simulink model "FourAGVsFullModel"  (R2019b)
settings: Solver=VariableStepAuto  StartTime=0.0  StopTime=200  RelTol=1e-3
values from neighbouring files (symbols this model uses):
  n = Datesize(1,1)    [AGVPlot.m]
undefined symbols (not defined in the file or in its folder): m, sigbuilder_block
settings Model: PacingRate=2  Creator=Khaled  LastModifiedBy=Khaled

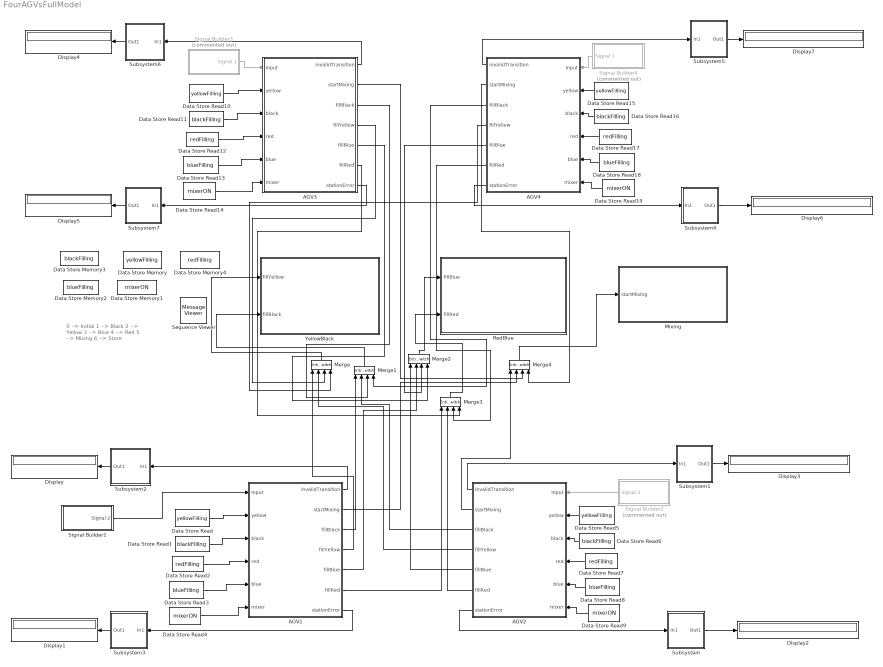
== system FourAGVsFullModel ==
  note: 0 --> Initial
      | 1 --> Black
      | 2 --> Yellow
      | 3 --> Blue
      | 4 --> Red
      | 5 --> Mixing
      | 6 --> Store
  AGV1 : Stateflow chart  BlockKeywords=__PRM__SERIALIZED__DATA__:Stateflow Chart,Stateflow Diagram  TreatAsAtomicUnit=on
  AGV2 : Stateflow chart  BlockKeywords=__PRM__SERIALIZED__DATA__:Stateflow Chart,Stateflow Diagram  TreatAsAtomicUnit=on
  AGV3 : Stateflow chart  BlockKeywords=__PRM__SERIALIZED__DATA__:Stateflow Chart,Stateflow Diagram  TreatAsAtomicUnit=on
  AGV4 : Stateflow chart  BlockKeywords=__PRM__SERIALIZED__DATA__:Stateflow Chart,Stateflow Diagram  TreatAsAtomicUnit=on
  Data Store Read{,5,10,15} (4 alike) : DataStoreRead  DataStoreName=yellowFilling
  Data Store Read{1,6,11,16} (4 alike) : DataStoreRead  DataStoreName=blackFilling
  Data Store Read{2,7,12,17} (4 alike) : DataStoreRead  DataStoreName=redFilling
  Data Store Read{3,8,13,18} (4 alike) : DataStoreRead  DataStoreName=blueFilling
  Data Store Read{4,9,14,19} (4 alike) : DataStoreRead  DataStoreName=mixerON
  Data Store Memory : DataStoreMemory  DataStoreName=yellowFilling  ReadBeforeWriteMsg=warning  WriteAfterWriteMsg=warning  WriteAfterReadMsg=warning  ShowAdditionalParam=off  OutDataTypeStr=double
  Data Store Memory1 : DataStoreMemory  DataStoreName=mixerON  ReadBeforeWriteMsg=warning  WriteAfterWriteMsg=warning  WriteAfterReadMsg=warning  ShowAdditionalParam=off  OutDataTypeStr=double
  Data Store Memory2 : DataStoreMemory  DataStoreName=blueFilling  ReadBeforeWriteMsg=warning  WriteAfterWriteMsg=warning  WriteAfterReadMsg=warning  ShowAdditionalParam=off  OutDataTypeStr=double
  Data Store Memory3 : DataStoreMemory  DataStoreName=blackFilling  ReadBeforeWriteMsg=warning  WriteAfterWriteMsg=warning  WriteAfterReadMsg=warning  ShowAdditionalParam=off  OutDataTypeStr=double
  Data Store Memory4 : DataStoreMemory  DataStoreName=redFilling  ReadBeforeWriteMsg=warning  WriteAfterWriteMsg=warning  WriteAfterReadMsg=warning  ShowAdditionalParam=off  OutDataTypeStr=double
  Display{,1..7} (8 alike) : Display
  Merge{,1..4} (5 alike) : EntityInputSwitch  InputPortMessageModes=m,m,m,m  OutputPortMessageModes=m  NumberInputPorts=4  SwitchingCriterion=From control port  InitialPortSelection=x
      settings: InputPortMap=u1,u2,u3,u4
  Mixing : Stateflow chart  BlockKeywords=__PRM__SERIALIZED__DATA__:Stateflow Chart,Stateflow Diagram  TreatAsAtomicUnit=on
  RedBlue : Stateflow chart  BlockKeywords=__PRM__SERIALIZED__DATA__:Stateflow Chart,Stateflow Diagram  TreatAsAtomicUnit=on
  Sequence Viewer : MessageViewer  VariableStepTimePrecision=16  ShowAllLifelines=off  AutoLayout=off  History=100  ShowMessages=off
  Signal Builder1 : Subsystem  Tag=STV Subsys  LoadFcn=sigbuilder_block('load');  StartFcn=sigbuilder_block('start');  StopFcn=sigbuilder_block('stop');  ClipboardFcn=sigbuilder_block('clipboard');  mask(Sigbuilder block){tuvar=[0:10]}
      mask help: Simulink:masks:SigbuilderBlock_MD
      mask init:
      | if ~strcmp(get_param(bdroot(gcbh),'SimulationStatus'),'stopped') tuvar = sigbuilder_block('maskInit'); end
      settings: CopyFcn=sigbuilder_block('copy');  DeleteFcn=sigbuilder_block('delete');  ModelCloseFcn=sigbuilder_block('modelClose');  PreSaveFcn=sigbuilder_block('preSave');  PauseFcn=sigbuilder_block('pause');  ContinueFcn=sigbuilder_block('continue');  NameChangeFcn=sigbuilder_block('namechange');  OpenFcn=sigbuilder_block('open',[5.4 30 1141.2 522.6 ]);  CloseFcn=sigbuilder_block('close');
      mask Display: plot(0, 0, 100, 100,[2, 2, 32, 32, 2], [68, 8, 8, 68, 68],[32, 2], [38, 38], [32, 19, 2],[53, 60, 44], [32, 17, 17, 2],[16, 16, 31, 31]);txt = getActiveGroup(gcbh);text(2, 100, txt,'verticalAlignment', 'top');
  Signal Builder2 : Subsystem  Tag=STV Subsys  Commented=on  LoadFcn=sigbuilder_block('load');  StartFcn=sigbuilder_block('start');  StopFcn=sigbuilder_block('stop');  ClipboardFcn=sigbuilder_block('clipboard');  mask(Sigbuilder block){tuvar=[0:10]}
      mask help: Simulink:masks:SigbuilderBlock_MD
      mask init:
      | if ~strcmp(get_param(bdroot(gcbh),'SimulationStatus'),'stopped') tuvar = sigbuilder_block('maskInit'); end
      settings: CopyFcn=sigbuilder_block('copy');  DeleteFcn=sigbuilder_block('delete');  ModelCloseFcn=sigbuilder_block('modelClose');  PreSaveFcn=sigbuilder_block('preSave');  PauseFcn=sigbuilder_block('pause');  ContinueFcn=sigbuilder_block('continue');  NameChangeFcn=sigbuilder_block('namechange');  OpenFcn=sigbuilder_block('open',[-61.2 14.4 1141.2 522.6 ]);  CloseFcn=sigbuilder_block('close');
      mask Display: plot(0, 0, 100, 100,[2, 2, 32, 32, 2], [68, 8, 8, 68, 68],[32, 2], [38, 38], [32, 19, 2],[53, 60, 44], [32, 17, 17, 2],[16, 16, 31, 31]);txt = getActiveGroup(gcbh);text(2, 100, txt,'verticalAlignment', 'top');
  Signal Builder3 : Subsystem  Tag=STV Subsys  Commented=on  LoadFcn=sigbuilder_block('load');  StartFcn=sigbuilder_block('start');  StopFcn=sigbuilder_block('stop');  ClipboardFcn=sigbuilder_block('clipboard');  mask(Sigbuilder block){tuvar=[0:10]}
      mask help: Simulink:masks:SigbuilderBlock_MD
      mask init:
      | if ~strcmp(get_param(bdroot(gcbh),'SimulationStatus'),'stopped') tuvar = sigbuilder_block('maskInit'); end
      settings: CopyFcn=sigbuilder_block('copy');  DeleteFcn=sigbuilder_block('delete');  ModelCloseFcn=sigbuilder_block('modelClose');  PreSaveFcn=sigbuilder_block('preSave');  PauseFcn=sigbuilder_block('pause');  ContinueFcn=sigbuilder_block('continue');  NameChangeFcn=sigbuilder_block('namechange');  OpenFcn=sigbuilder_block('open',[303.6 76.2 579.6 400.2 ]);  CloseFcn=sigbuilder_block('close');
      mask Display: plot(0, 0, 100, 100,[2, 2, 32, 32, 2], [68, 8, 8, 68, 68],[32, 2], [38, 38], [32, 19, 2],[53, 60, 44], [32, 17, 17, 2],[16, 16, 31, 31]);txt = getActiveGroup(gcbh);text(2, 100, txt,'verticalAlignment', 'top');
  Signal Builder4 : Subsystem  Tag=STV Subsys  Commented=on  LoadFcn=sigbuilder_block('load');  StartFcn=sigbuilder_block('start');  StopFcn=sigbuilder_block('stop');  ClipboardFcn=sigbuilder_block('clipboard');  mask(Sigbuilder block){tuvar=[0:10]}
      mask help: Simulink:masks:SigbuilderBlock_MD
      mask init:
      | if ~strcmp(get_param(bdroot(gcbh),'SimulationStatus'),'stopped') tuvar = sigbuilder_block('maskInit'); end
      settings: CopyFcn=sigbuilder_block('copy');  DeleteFcn=sigbuilder_block('delete');  ModelCloseFcn=sigbuilder_block('modelClose');  PreSaveFcn=sigbuilder_block('preSave');  PauseFcn=sigbuilder_block('pause');  ContinueFcn=sigbuilder_block('continue');  NameChangeFcn=sigbuilder_block('namechange');  OpenFcn=sigbuilder_block('open',[440.4 98.4 579.6 400.2 ]);  CloseFcn=sigbuilder_block('close');
      mask Display: plot(0, 0, 100, 100,[2, 2, 32, 32, 2], [68, 8, 8, 68, 68],[32, 2], [38, 38], [32, 19, 2],[53, 60, 44], [32, 17, 17, 2],[16, 16, 31, 31]);txt = getActiveGroup(gcbh);text(2, 100, txt,'verticalAlignment', 'top');
  Subsystem : Subsystem
  Subsystem1 : Subsystem
  Subsystem2 : Subsystem
  Subsystem3 : Subsystem
  Subsystem4 : Subsystem
  Subsystem5 : Subsystem
  Subsystem6 : Subsystem
  Subsystem7 : Subsystem
  YellowBlack : Stateflow chart  BlockKeywords=__PRM__SERIALIZED__DATA__:Stateflow Chart,Stateflow Diagram  TreatAsAtomicUnit=on
  wires:
  AGV3/6(fillRed) -> Merge3/4
  Data Store Read5/1 -> AGV2/2(yellow)
  Data Store Read18/1 -> AGV4/5(blue)
  AGV3/2(startMixing) -> Merge4/3
  AGV3/1(invalidTransition) -> Subsystem6/1(In1)
  Data Store Read6/1 -> AGV2/3(black)
  AGV3/3(fillBlack) -> Merge1/3
  Data Store Read19/1 -> AGV4/6(mixer)
  Data Store Read14/1 -> AGV3/6(mixer)
  Data Store Read12/1 -> AGV3/4(red)
  AGV4/2(startMixing) -> Merge4/4
  Subsystem5/1(Out1) -> Display7/1
  AGV3/4(fillYellow) -> Merge/3
  Merge4/1 -> Mixing/1(startMixing)
  AGV3/7(stationError) -> Subsystem7/1(In1)
  Data Store Read8/1 -> AGV2/5(blue)
  Data Store Read13/1 -> AGV3/5(blue)
  Signal Builder3/1(Signal 1) -> AGV3/1(Input)
  AGV1/6(fillRed) -> Merge3/1
  AGV4/7(stationError) -> Subsystem4/1(In1)
  Data Store Read11/1 -> AGV3/3(black)
  Subsystem7/1(Out1) -> Display5/1
  Signal Builder4/1(Signal 1) -> AGV4/1(Input)
  Subsystem4/1(Out1) -> Display6/1
  AGV3/5(fillBlue) -> Merge2/4
  Data Store Read4/1 -> AGV1/6(mixer)
  Data Store Read17/1 -> AGV4/4(red)
  Data Store Read16/1 -> AGV4/3(black)
  AGV2/2(startMixing) -> Merge4/1
  AGV4/6(fillRed) -> Merge3/3
  Data Store Read15/1 -> AGV4/2(yellow)
  AGV1/1(invalidTransition) -> Subsystem2/1(In1)
  Data Store Read7/1 -> AGV2/4(red)
  Signal Builder2/1(Signal 2) -> AGV2/1(Input)
  AGV2/1(invalidTransition) -> Subsystem1/1(In1)
  Subsystem1/1(Out1) -> Display3/1
  AGV2/7(stationError) -> Subsystem/1(In1)
  Subsystem6/1(Out1) -> Display4/1
  Subsystem3/1(Out1) -> Display1/1
  AGV4/5(fillBlue) -> Merge2/3
  AGV2/5(fillBlue) -> Merge2/1
  AGV1/7(stationError) -> Subsystem3/1(In1)
  AGV1/5(fillBlue) -> Merge2/2
  Subsystem2/1(Out1) -> Display/1
  Data Store Read10/1 -> AGV3/2(yellow)
  Data Store Read1/1 -> AGV1/3(black)
  AGV1/3(fillBlack) -> Merge1/1
  Data Store Read9/1 -> AGV2/6(mixer)
  Merge3/1 -> RedBlue/2(fillRed)
  Merge/1 -> YellowBlack/1(fillYellow)
  AGV1/2(startMixing) -> Merge4/2
  AGV4/3(fillBlack) -> Merge1/4
  AGV2/3(fillBlack) -> Merge1/2
  AGV4/1(invalidTransition) -> Subsystem5/1(In1)
  Merge1/1 -> YellowBlack/2(fillBlack)
  Merge2/1 -> RedBlue/1(fillBlue)
  AGV2/6(fillRed) -> Merge3/2
  AGV4/4(fillYellow) -> Merge/4
  Data Store Read/1 -> AGV1/2(yellow)
  Data Store Read3/1 -> AGV1/5(blue)
  AGV2/4(fillYellow) -> Merge/2
  Subsystem/1(Out1) -> Display2/1
  AGV1/4(fillYellow) -> Merge/1
  Data Store Read2/1 -> AGV1/4(red)
  Signal Builder1/1(Signal 2) -> AGV1/1(Input)

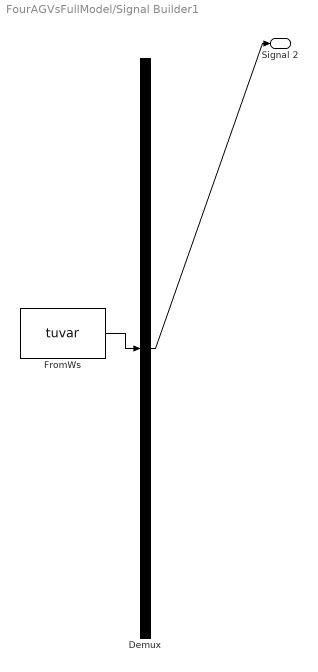
== system FourAGVsFullModel/Signal Builder1 ==
  Demux : Demux  Tag=STV Demux  Outputs=1
  FromWs : FromWorkspace  Tag=STV FromWs  VariableName=tuvar  SampleTime=0
      SigBuilderData=|
      | common.afterFinalStr = 'Extrapolate'
      | common.sampleTime = 0
      | dataSet.timeRange = [0 345]
      | dataSet.name = 'Group 1'
      | sbobj.Groups.Name = 'Group 1'
      | sbobj.Groups.Signals.Name = 'Signal 2'
      | sbobj.Groups.Signals.XData = [0 30 30 60 60 80 80 105 105 150 150 185 185 195 195 225 225 245 245 300 300 309.5 314.5 317 320.5 325 329 333 335 335 338.5 341.5 345]
      | sbobj.Groups.Signals.YData = [0 0 6 6 1 1 3 3 5 5 6 6 0 0 6 6 2 2 5 5 6 6 6 6 6 6 6 6 6 0 0 0 0]
      | sbobj.Groups.TimeRange = [0 345]
  Signal 2 : Outport  Tag=STV Outport
  wires:
  FromWs/1 -> Demux/1
  Demux/1 -> Signal 2/1

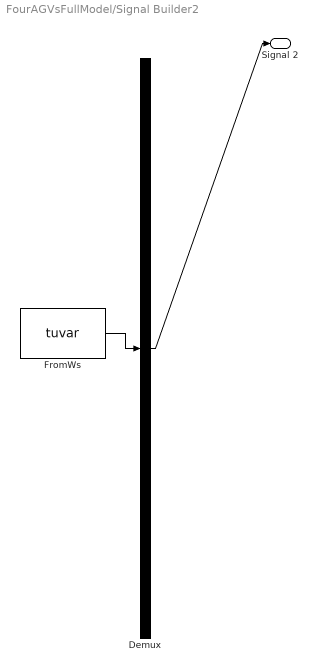
== system FourAGVsFullModel/Signal Builder2 ==
  Demux : Demux  Tag=STV Demux  Outputs=1
  FromWs : FromWorkspace  Tag=STV FromWs  VariableName=tuvar  SampleTime=0
      SigBuilderData=|
      | common.afterFinalStr = 'Extrapolate'
      | common.sampleTime = 0
      | dataSet.timeRange = [0 400]
      | dataSet.name = 'Group 1'
      | sbobj.Groups.Name = 'Group 1'
      | sbobj.Groups.Signals.Name = 'Signal 2'
      | sbobj.Groups.Signals.XData = [0 30 30 50 50 75 75 110 110 120 120 150 150 180 180 225 225 260 260 270 270 300 300 320 320 332 340 345 345 358 366 371.5 380 380 400]
      | sbobj.Groups.Signals.YData = [6 6 3 3 5 5 6 6 0 0 6 6 2 2 5 5 6 6 0 0 6 6 4 4 5 5 5 5 6 6 6 6 6 0 0]
      | sbobj.Groups.TimeRange = [0 400]
  Signal 2 : Outport  Tag=STV Outport
  wires:
  FromWs/1 -> Demux/1
  Demux/1 -> Signal 2/1

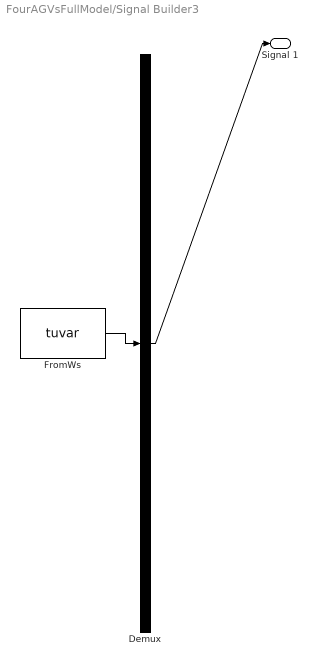
== system FourAGVsFullModel/Signal Builder3 ==
  Demux : Demux  Tag=STV Demux  Outputs=1
  FromWs : FromWorkspace  Tag=STV FromWs  VariableName=tuvar  SampleTime=0
      SigBuilderData=|
      | common.afterFinalStr = 'Extrapolate'
      | common.sampleTime = 0
      | dataSet.timeRange = [0 100]
      | dataSet.name = 'Group 1'
      | sbobj.Groups.Name = 'Group 1'
      | sbobj.Groups.Signals.Name = 'Signal 1'
      | sbobj.Groups.Signals.XData = [0 23 23 46 46 66 66 87.5 87.5 93.75 100]
      | sbobj.Groups.Signals.YData = [2 2 4 4 5 5 6 6 0 0 0]
      | sbobj.Groups.TimeRange = [0 100]
  Signal 1 : Outport  Tag=STV Outport
  wires:
  FromWs/1 -> Demux/1
  Demux/1 -> Signal 1/1

== system FourAGVsFullModel/Signal Builder4 ==
  Demux : Demux  Tag=STV Demux  Outputs=1
  FromWs : FromWorkspace  Tag=STV FromWs  VariableName=tuvar  SampleTime=0
      SigBuilderData=|
      | common.afterFinalStr = 'Extrapolate'
      | common.sampleTime = 0
      | dataSet.timeRange = [0 100]
      | dataSet.name = 'Group 1'
      | sbobj.Groups.Name = 'Group 1'
      | sbobj.Groups.Signals.Name = 'Signal 1'
      | sbobj.Groups.Signals.XData = [0 23 23 46 66 66 87.5 87.5 93.75 100]
      | sbobj.Groups.Signals.YData = [0 0 4 4 4 5 5 0 0 0]
      | sbobj.Groups.TimeRange = [0 100]
  Signal 1 : Outport  Tag=STV Outport
  wires:
  FromWs/1 -> Demux/1
  Demux/1 -> Signal 1/1

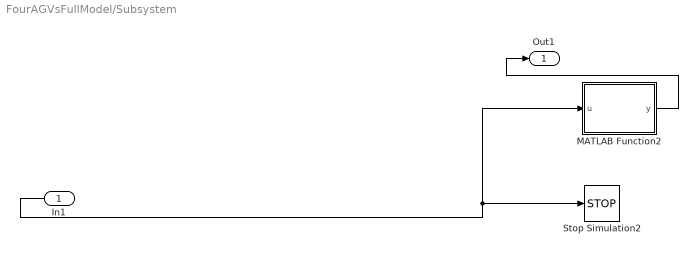
== system FourAGVsFullModel/Subsystem ==
  In1 : Inport
  MATLAB Function2 : MATLAB Function  TreatAsAtomicUnit=on
  Stop Simulation2 : Stop
  Out1 : Outport
  wires:
  In1/1 -> MATLAB Function2/1(u), Stop Simulation2/1
  MATLAB Function2/1(y) -> Out1/1

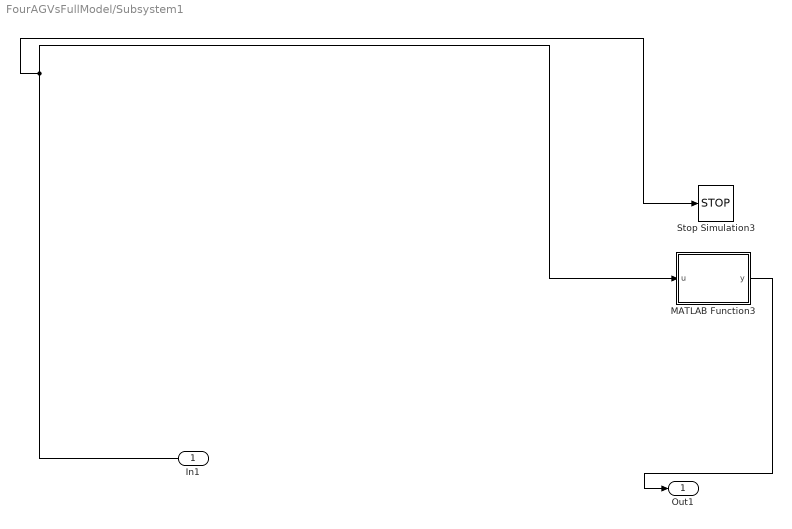
== system FourAGVsFullModel/Subsystem1 ==
  In1 : Inport
  MATLAB Function3 : MATLAB Function  TreatAsAtomicUnit=on
  Stop Simulation3 : Stop
  Out1 : Outport
  wires:
  In1/1 -> Stop Simulation3/1, MATLAB Function3/1(u)
  MATLAB Function3/1(y) -> Out1/1

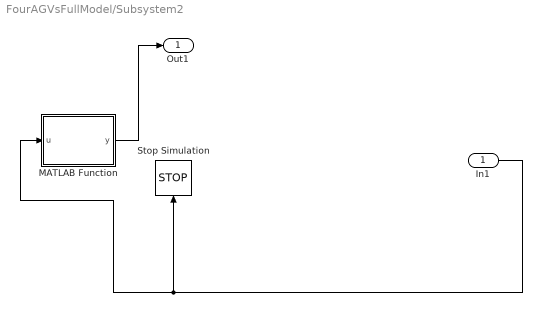
== system FourAGVsFullModel/Subsystem2 ==
  In1 : Inport
  MATLAB Function : MATLAB Function  TreatAsAtomicUnit=on
  Stop Simulation : Stop
  Out1 : Outport
  wires:
  MATLAB Function/1(y) -> Out1/1
  In1/1 -> MATLAB Function/1(u), Stop Simulation/1

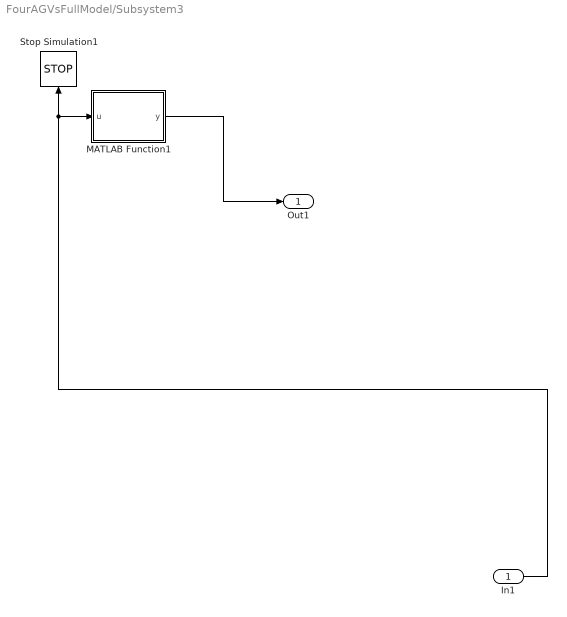
== system FourAGVsFullModel/Subsystem3 ==
  In1 : Inport
  MATLAB Function1 : MATLAB Function  TreatAsAtomicUnit=on
  Stop Simulation1 : Stop
  Out1 : Outport
  wires:
  In1/1 -> Stop Simulation1/1, MATLAB Function1/1(u)
  MATLAB Function1/1(y) -> Out1/1

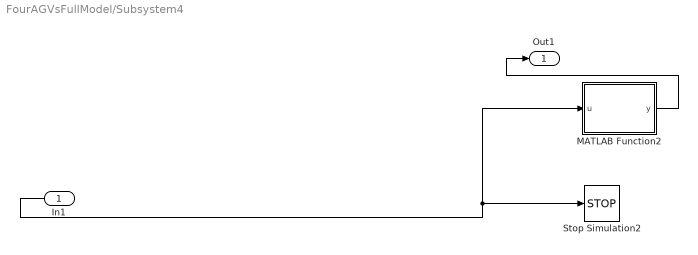
== system FourAGVsFullModel/Subsystem4 ==
  In1 : Inport
  MATLAB Function2 : MATLAB Function  TreatAsAtomicUnit=on
  Stop Simulation2 : Stop
  Out1 : Outport
  wires:
  In1/1 -> MATLAB Function2/1(u), Stop Simulation2/1
  MATLAB Function2/1(y) -> Out1/1

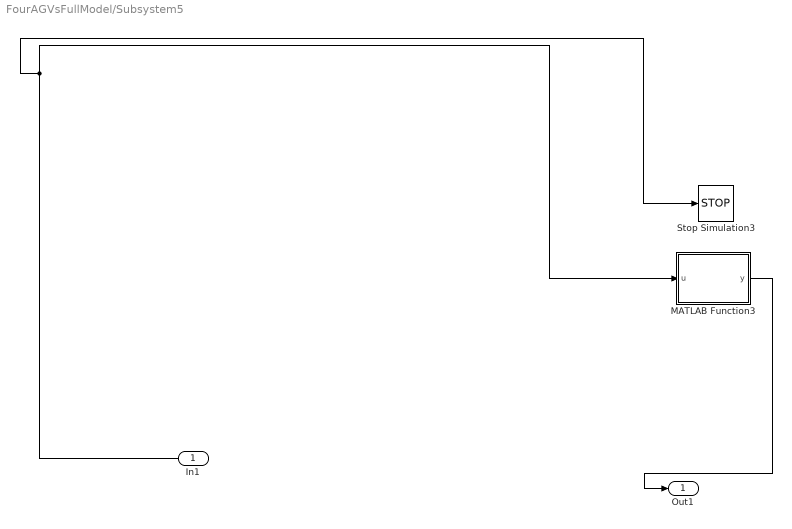
== system FourAGVsFullModel/Subsystem5 ==
  In1 : Inport
  MATLAB Function3 : MATLAB Function  TreatAsAtomicUnit=on
  Stop Simulation3 : Stop
  Out1 : Outport
  wires:
  In1/1 -> Stop Simulation3/1, MATLAB Function3/1(u)
  MATLAB Function3/1(y) -> Out1/1

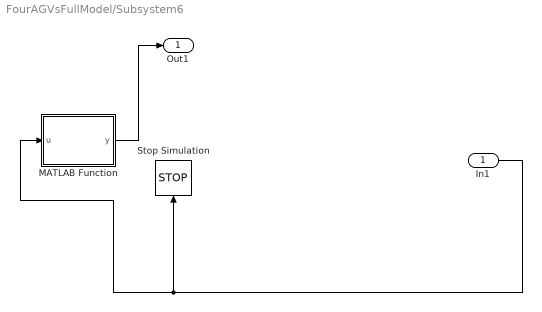
== system FourAGVsFullModel/Subsystem6 ==
  In1 : Inport
  MATLAB Function : MATLAB Function  TreatAsAtomicUnit=on
  Stop Simulation : Stop
  Out1 : Outport
  wires:
  MATLAB Function/1(y) -> Out1/1
  In1/1 -> MATLAB Function/1(u), Stop Simulation/1

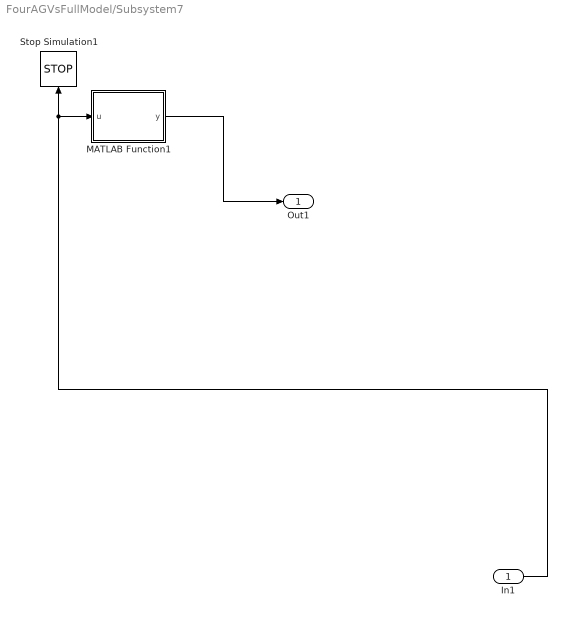
== system FourAGVsFullModel/Subsystem7 ==
  In1 : Inport
  MATLAB Function1 : MATLAB Function  TreatAsAtomicUnit=on
  Stop Simulation1 : Stop
  Out1 : Outport
  wires:
  In1/1 -> Stop Simulation1/1, MATLAB Function1/1(u)
  MATLAB Function1/1(y) -> Out1/1

== stateflow chart FourAGVsFullModel/AGV1 ==
  state Black
    en:
    send(fillBlack);
  state Yellow
    en:
    send(fillYellow);
  state YBToMixing
  state YBToRB
  state StorageToYB
  state StationErrorState
    stationError=1;
  state MixingStation
    en:
    send(startMixing);
  state Storage
  state InvalidTransitionState
    invalidTransition=1;
  state StorageToInit
  state InitToStorage
  state MixingToStorage
  state InitPosition
  state RBToYB
  state RBToMixing
  state StorageToRB
  state Red
    en:
    send(fillRed);
  state Blue
    en:
    send(fillBlue);
  Yellow -> YBToMixing [order 4] : [Input==5]
  Yellow -> YBToRB [order 3] : [Input==3 || Input==4]
  Yellow -> Black [order 1] : [Input==1]
  (junction 173) -> Yellow [order 1] : [black==0 && yellow==0]
  StorageToYB -> (junction 173) [order 2] : [Input==2 && after(T_S_YB,sec)]
  Black -> Yellow [order 1] : [Input==2]
  RBToYB -> (junction 173) [order 1] : [Input==2 && ...
      | after(T_RB_YB,sec)]
  (junction 173) -> StationErrorState [order 2] : [black==1 || yellow==1]
  StorageToYB -> (junction 176) [order 1] : [Input==1 && ...
      | after(T_S_YB,sec)]
  (junction 176) -> Black [order 1] : [black==0 && yellow==0]
  Black -> YBToMixing [order 4] : [Input==5]
  RBToYB -> (junction 176) [order 2] : [Input==1 && ...
      | after(T_RB_YB,sec)]
  Black -> InvalidTransitionState [order 3] : [Input==6 || Input==0]
  Black -> YBToRB [order 2] : [Input==3 || Input==4]
  Yellow -> InvalidTransitionState [order 2] : [Input==6 || Input==0]
  (junction 176) -> StationErrorState [order 2] : [black==1 || yellow==1]
  YBToMixing -> (junction 185) : [Input==5 && after(T_YB_M,sec)]
  YBToRB -> (junction 182) [order 2] : [Input==4 && ...
      | after(T_YB_RB,sec)]
  YBToRB -> (junction 179) [order 1] : [Input==3 && ...
      | after(T_YB_RB,sec)]
  Storage -> Storage [order 5] : [Input==6]
  Storage -> StorageToYB [order 1] : [Input==1 || Input==2]
  (junction 185) -> MixingStation [order 1] : [mixer==0]
  (junction 185) -> StationErrorState [order 2] : [mixer==1]
  Storage -> StorageToRB [order 3] : [Input==3 || Input==4]
  (junction 182) -> StationErrorState [order 2] : [blue==1 || red==1]
  RBToMixing -> (junction 185) : [Input==5 && ...
      |  after(T_RB_M,sec)]
  Storage -> InvalidTransitionState [order 4] : [Input==5]
  (junction 179) -> StationErrorState [order 2] : [blue==1 || red==1]
  MixingStation -> InvalidTransitionState [order 1] : [Input==0 ||Input==1 ||Input==2 ...
      | || Input==3 ||Input==4 ]
  InitToStorage -> Storage : after(T_Init_S,sec)
  MixingStation -> MixingToStorage [order 2] : [Input==6]
  MixingToStorage -> Storage : [Input==6 && after(T_M_S,sec)]
  Storage -> StorageToInit [order 2] : [Input==0]
  InitPosition -> InvalidTransitionState [order 3] : [Input==5 ]
  Red -> InvalidTransitionState [order 2] : [Input==6 || Input==0]
  Blue -> InvalidTransitionState [order 3] : [Input==6 || Input==0]
  StorageToInit -> InitPosition : after(T_Init_S,sec)
  InitPosition -> InitToStorage [order 1] : [Input==1 || Input==2 || Input==3 || Input==4|| Input==6]
  (default) -> InitPosition
  Red -> RBToYB [order 4] : [Input==2 || Input==1]
  Blue -> RBToYB [order 2] : [Input==1 || Input==2]
  InitPosition -> InitPosition [order 2] : [Input==0]
  StorageToRB -> StorageToRB [order 3] : [Input==3 || Input==4]
  Blue -> RBToMixing [order 4] : [Input==5]
  Red -> RBToMixing [order 3] : [Input==5]
  StorageToRB -> (junction 182) [order 2] : [Input==4 &&...
      |  after(T_S_RB,sec)]
  (junction 182) -> Red [order 1] : [blue==0&&red==0]
  StorageToRB -> (junction 179) [order 1] : [Input==3 && after(T_S_RB,sec)]
  (junction 179) -> Blue [order 1] : [blue==0&&red==0]
  Blue -> Red [order 1] : [Input==4]
  Red -> Blue [order 1] : [Input==3]
  data: Input input; invalidTransition output; startMixing output boolean size=1; fillBlack output boolean size=1; fillYellow output boolean size=1; fillBlue output boolean size=1; fillRed output boolean size=1; yellow input; black input; red input; blue input; mixer input; stationError output; T_YB_M constant double =10; T_RB_YB constant double =15; T_RB_M constant double =10; T_S_YB constant double =10; T_S_RB constant double =10; T_YB_RB constant double =15; T_M_S constant double =15; T_Init_S constant double =10

== matlab function FourAGVsFullModel/Subsystem2/MATLAB Function ==
  data: u input; y output string
function y= fcn(u)
if(u==1)
    y="Invalid Transition";
else
    y="No Error";
end

== stateflow chart FourAGVsFullModel/Mixing ==
  state MixerOFF
    mixerON=0;
  state MixerON
    mixerON=1;
  MixerOFF -> MixerON : startMixing
  (default) -> MixerOFF
  MixerON -> MixerOFF : after(15,sec)
  data: startMixing input; mixerON data_store_memory

== matlab function FourAGVsFullModel/Subsystem3/MATLAB Function1 ==
  data: u input; y output string
function y= fcn(u)
if(u==1)
    y="station is busy";
else
    y="No Error";
end

== stateflow chart FourAGVsFullModel/YellowBlack ==
  state Nofilling
    yellowFilling=0;
    blackFilling=0;
  state fillingBlack
    blackFilling=1;
  state FillingYellow
    yellowFilling=1;
  (default) -> Nofilling
  Nofilling -> fillingBlack [order 1] : fillBlack
  Nofilling -> FillingYellow [order 2] : fillYellow
  fillingBlack -> Nofilling : after(10,sec)
  FillingYellow -> Nofilling : after(10,sec)
  data: fillYellow input; fillBlack input; yellowFilling data_store_memory; blackFilling data_store_memory

== stateflow chart FourAGVsFullModel/RedBlue ==
  state Nofilling
    blueFilling=0;
    redFilling=0;
  state FillingRed
    redFilling=1;
  state FillingBlue
    blueFilling=1;
  (default) -> Nofilling
  Nofilling -> FillingRed [order 1] : fillRed
  Nofilling -> FillingBlue [order 2] : fillBlue
  FillingRed -> Nofilling : after(10,sec)
  FillingBlue -> Nofilling : after(10,sec)
  data: fillBlue input; fillRed input; blueFilling data_store_memory; redFilling data_store_memory

== stateflow chart FourAGVsFullModel/AGV2 ==
  state Black
    en:
    send(fillBlack);
  state Yellow
    en:
    send(fillYellow);
  state YBToMixing
  state YBToRB
  state StorageToYB
  state StationErrorState
    stationError=1;
  state MixingStation
    en:
    send(startMixing);
  state Storage
  state InvalidTransitionState
    invalidTransition=1;
  state StorageToInit
  state InitToStorage
  state MixingToStorage
  state InitPosition
  state RBToYB
  state RBToMixing
  state StorageToRB
  state Red
    en:
    send(fillRed);
  state Blue
    en:
    send(fillBlue);
  Yellow -> YBToMixing [order 4] : [Input==5]
  Yellow -> YBToRB [order 3] : [Input==3 || Input==4]
  Yellow -> Black [order 1] : [Input==1]
  (junction 173) -> Yellow [order 1] : [black==0 && yellow==0]
  StorageToYB -> (junction 173) [order 2] : [Input==2 && after(T_S_YB,sec)]
  Black -> Yellow [order 1] : [Input==2]
  RBToYB -> (junction 173) [order 1] : [Input==2 && ...
      | after(T_RB_YB,sec)]
  (junction 173) -> StationErrorState [order 2] : [black==1 || yellow==1]
  StorageToYB -> (junction 176) [order 1] : [Input==1 && ...
      | after(T_S_YB,sec)]
  (junction 176) -> Black [order 1] : [black==0 && yellow==0]
  Black -> YBToMixing [order 4] : [Input==5]
  RBToYB -> (junction 176) [order 2] : [Input==1 && ...
      | after(T_RB_YB,sec)]
  Black -> InvalidTransitionState [order 3] : [Input==6 || Input==0]
  Black -> YBToRB [order 2] : [Input==3 || Input==4]
  Yellow -> InvalidTransitionState [order 2] : [Input==6 || Input==0]
  (junction 176) -> StationErrorState [order 2] : [black==1 || yellow==1]
  YBToMixing -> (junction 185) : [Input==5 && after(T_YB_M,sec)]
  YBToRB -> (junction 182) [order 2] : [Input==4 && ...
      | after(T_YB_RB,sec)]
  YBToRB -> (junction 179) [order 1] : [Input==3 && ...
      | after(T_YB_RB,sec)]
  Storage -> Storage [order 5] : [Input==6]
  Storage -> StorageToYB [order 1] : [Input==1 || Input==2]
  (junction 185) -> MixingStation [order 1] : [mixer==0]
  (junction 185) -> StationErrorState [order 2] : [mixer==1]
  Storage -> StorageToRB [order 3] : [Input==3 || Input==4]
  (junction 182) -> StationErrorState [order 2] : [blue==1 || red==1]
  RBToMixing -> (junction 185) : [Input==5 && ...
      |  after(T_RB_M,sec)]
  Storage -> InvalidTransitionState [order 4] : [Input==5]
  (junction 179) -> StationErrorState [order 2] : [blue==1 || red==1]
  MixingStation -> InvalidTransitionState [order 1] : [Input==0 ||Input==1 ||Input==2 ...
      | || Input==3 ||Input==4 ]
  InitToStorage -> Storage : after(T_Init_S,sec)
  MixingStation -> MixingToStorage [order 2] : [Input==6]
  MixingToStorage -> Storage : [Input==6 && after(T_M_S,sec)]
  Storage -> StorageToInit [order 2] : [Input==0]
  InitPosition -> InvalidTransitionState [order 3] : [Input==5 ]
  Red -> InvalidTransitionState [order 2] : [Input==6 || Input==0]
  Blue -> InvalidTransitionState [order 3] : [Input==6 || Input==0]
  StorageToInit -> InitPosition : after(T_Init_S,sec)
  InitPosition -> InitToStorage [order 1] : [Input==1 || Input==2 || Input==3 || Input==4|| Input==6]
  (default) -> InitPosition
  Red -> RBToYB [order 4] : [Input==2 || Input==1]
  Blue -> RBToYB [order 2] : [Input==1 || Input==2]
  InitPosition -> InitPosition [order 2] : [Input==0]
  Blue -> RBToMixing [order 4] : [Input==5]
  Red -> RBToMixing [order 3] : [Input==5]
  StorageToRB -> (junction 182) [order 2] : [Input==4 &&...
      |  after(T_S_RB,sec)]
  (junction 182) -> Red [order 1] : [blue==0&&red==0]
  StorageToRB -> (junction 179) [order 1] : [Input==3 && after(T_S_RB,sec)]
  (junction 179) -> Blue [order 1] : [blue==0&&red==0]
  Blue -> Red [order 1] : [Input==4]
  Red -> Blue [order 1] : [Input==3]
  data: Input input; invalidTransition output; startMixing output boolean size=1; fillBlack output boolean size=1; fillYellow output boolean size=1; fillBlue output boolean size=1; fillRed output boolean size=1; yellow input; black input; red input; blue input; mixer input; stationError output; T_YB_M constant double =10; T_RB_YB constant double =15; T_RB_M constant double =10; T_S_YB constant double =10; T_S_RB constant double =10; T_YB_RB constant double =15; T_M_S constant double =15; T_Init_S constant double =10

== matlab function FourAGVsFullModel/Subsystem/MATLAB Function2 ==
  data: u input; y output string
function y= fcn(u)
if(u==1)
    y="station is busy";
else
    y="No Error";
end

== matlab function FourAGVsFullModel/Subsystem1/MATLAB Function3 ==
  data: u input; y output string
function y= fcn(u)
if(u==1)
    y="station is busy";
else
    y="No Error";
end

== stateflow chart FourAGVsFullModel/AGV3 ==
  state Black
    en:
    send(fillBlack);
  state Yellow
    en:
    send(fillYellow);
  state YBToMixing
  state YBToRB
  state StorageToYB
  state StationErrorState
    stationError=1;
  state MixingStation
    en:
    send(startMixing);
  state Storage
  state Transition
  state InvalidTransitionState
    invalidTransition=1;
  state StorageToInit
  state MixingToStorage
  state InitPosition
  state RBToYB
  state RBToMixing
  state StorageToRB
  state Red
    en:
    send(fillRed);
  state Blue
    en:
    send(fillBlue);
  Yellow -> YBToMixing [order 4] : [Input==5]
  Yellow -> YBToRB [order 3] : [Input==3 || Input==4]
  Yellow -> Black [order 1] : [Input==1]
  (junction 173) -> Yellow [order 1] : [black==0 && yellow==0]
  StorageToYB -> (junction 173) [order 2] : [Input==2 && after(T_S_YB,sec)]
  Black -> Yellow [order 1] : [Input==2]
  RBToYB -> (junction 173) [order 1] : [Input==2 && ...
      | after(T_RB_YB,sec)]
  (junction 173) -> StationErrorState [order 2] : [black==1 || yellow==1]
  StorageToYB -> (junction 176) [order 1] : [Input==1 && ...
      | after(T_S_YB,sec)]
  (junction 176) -> Black [order 1] : [black==0 && yellow==0]
  Black -> YBToMixing [order 4] : [Input==5]
  RBToYB -> (junction 176) [order 2] : [Input==1 && ...
      | after(T_RB_YB,sec)]
  Black -> InvalidTransitionState [order 3] : [Input==6 || Input==0]
  Black -> YBToRB [order 2] : [Input==3 || Input==4]
  Yellow -> InvalidTransitionState [order 2] : [Input==6 || Input==0]
  (junction 176) -> StationErrorState [order 2] : [black==1 || yellow==1]
  YBToMixing -> (junction 185) : [Input==5 && after(T_YB_M,sec)]
  YBToRB -> (junction 182) [order 2] : [Input==4 && ...
      | after(T_YB_RB,sec)]
  YBToRB -> (junction 179) [order 1] : [Input==3 && ...
      | after(T_YB_RB,sec)]
  Storage -> Storage [order 5] : [Input==6]
  Storage -> StorageToYB [order 1] : [Input==1 || Input==2]
  (junction 185) -> MixingStation [order 1] : [mixer==0]
  (junction 185) -> StationErrorState [order 2] : [mixer==1]
  Storage -> StorageToRB [order 3] : [Input==3 || Input==4]
  (junction 182) -> StationErrorState [order 2] : [blue==1 || red==1]
  RBToMixing -> (junction 185) : [Input==5 && ...
      |  after(T_RB_M,sec)]
  Storage -> InvalidTransitionState [order 4] : [Input==5]
  Transition -> Storage : after(time,sec)
  (junction 179) -> StationErrorState [order 2] : [blue==1 || red==1]
  MixingStation -> InvalidTransitionState [order 1] : [Input==0 ||Input==1 ||Input==2 ...
      | || Input==3 ||Input==4 ]
  MixingStation -> MixingToStorage [order 2] : [Input==6]
  MixingToStorage -> Storage : [Input==6 && after(T_M_S,sec)]
  Storage -> StorageToInit [order 2] : [Input==0]
  InitPosition -> InvalidTransitionState [order 3] : [Input==5 ]
  InitPosition -> Transition [order 1] : [Input==1 || Input==2 || Input==3 || Input==4|| Input==6]/{time=T_Init_S}
  Red -> InvalidTransitionState [order 2] : [Input==6 || Input==0]
  Blue -> InvalidTransitionState [order 3] : [Input==6 || Input==0]
  StorageToInit -> InitPosition : after(T_Init_S,sec)
  (default) -> InitPosition
  Red -> RBToYB [order 4] : [Input==2 || Input==1]
  Blue -> RBToYB [order 2] : [Input==1 || Input==2]
  InitPosition -> InitPosition [order 2] : [Input==0]
  Blue -> RBToMixing [order 4] : [Input==5]
  Red -> RBToMixing [order 3] : [Input==5]
  StorageToRB -> (junction 182) [order 2] : [Input==4 &&...
      |  after(T_S_RB,sec)]
  (junction 182) -> Red [order 1] : [blue==0&&red==0]
  StorageToRB -> (junction 179) [order 1] : [Input==3 && after(T_S_RB,sec)]
  (junction 179) -> Blue [order 1] : [blue==0&&red==0]
  Blue -> Red [order 1] : [Input==4]
  Red -> Blue [order 1] : [Input==3]
  data: Input input; invalidTransition output; startMixing output boolean size=1; fillBlack output boolean size=1; fillYellow output boolean size=1; fillBlue output boolean size=1; fillRed output boolean size=1; yellow input; black input; red input; blue input; mixer input; stationError output; T_YB_M constant double =10; T_RB_YB constant double =15; T_RB_M constant double =10; T_S_YB constant double =10; T_S_RB constant double =10; T_YB_RB constant double =15; T_M_S constant double =15; T_Init_S constant double =10; time local

== stateflow chart FourAGVsFullModel/AGV4 ==
  state Black
    en:
    send(fillBlack);
  state Yellow
    en:
    send(fillYellow);
  state YBToMixing
  state YBToRB
  state StorageToYB
  state StationErrorState
    stationError=1;
  state MixingStation
    en:
    send(startMixing);
  state Storage
  state InvalidTransitionState
    invalidTransition=1;
  state StorageToInit
  state InitToStorage
  state MixingToStorage
  state InitPosition
  state RBToYB
  state RBToMixing
  state StorageToRB
  state Red
    en:
    send(fillRed);
  state Blue
    en:
    send(fillBlue);
  Yellow -> YBToMixing [order 4] : [Input==5]
  Yellow -> YBToRB [order 3] : [Input==3 || Input==4]
  Yellow -> Black [order 1] : [Input==1]
  (junction 173) -> Yellow [order 1] : [black==0 && yellow==0]
  StorageToYB -> (junction 173) [order 2] : [Input==2 && after(T_S_YB,sec)]
  Black -> Yellow [order 1] : [Input==2]
  RBToYB -> (junction 173) [order 1] : [Input==2 && ...
      | after(T_RB_YB,sec)]
  (junction 173) -> StationErrorState [order 2] : [black==1 || yellow==1]
  StorageToYB -> (junction 176) [order 1] : [Input==1 && ...
      | after(T_S_YB,sec)]
  (junction 176) -> Black [order 1] : [black==0 && yellow==0]
  Black -> YBToMixing [order 4] : [Input==5]
  RBToYB -> (junction 176) [order 2] : [Input==1 && ...
      | after(T_RB_YB,sec)]
  Black -> InvalidTransitionState [order 3] : [Input==6 || Input==0]
  Black -> YBToRB [order 2] : [Input==3 || Input==4]
  Yellow -> InvalidTransitionState [order 2] : [Input==6 || Input==0]
  (junction 176) -> StationErrorState [order 2] : [black==1 || yellow==1]
  YBToMixing -> (junction 185) : [Input==5 && after(T_YB_M,sec)]
  YBToRB -> (junction 182) [order 2] : [Input==4 && ...
      | after(T_YB_RB,sec)]
  YBToRB -> (junction 179) [order 1] : [Input==3 && ...
      | after(T_YB_RB,sec)]
  Storage -> Storage [order 5] : [Input==6]
  Storage -> StorageToYB [order 1] : [Input==1 || Input==2]
  (junction 185) -> MixingStation [order 1] : [mixer==0]
  (junction 185) -> StationErrorState [order 2] : [mixer==1]
  Storage -> StorageToRB [order 3] : [Input==3 || Input==4]
  (junction 182) -> StationErrorState [order 2] : [blue==1 || red==1]
  RBToMixing -> (junction 185) : [Input==5 && ...
      |  after(T_RB_M,sec)]
  MixingStation -> InvalidTransitionState [order 1] : [Input==0 ||Input==1 ||Input==2 ...
      | || Input==3 ||Input==4 ]
  Storage -> InvalidTransitionState [order 4] : [Input==5]
  (junction 179) -> StationErrorState [order 2] : [blue==1 || red==1]
  InitToStorage -> Storage : after(T_Init_S,sec)
  MixingStation -> MixingToStorage [order 2] : [Input==6]
  MixingToStorage -> Storage : [Input==6 && after(T_M_S,sec)]
  Storage -> StorageToInit [order 2] : [Input==0]
  InitPosition -> InvalidTransitionState [order 3] : [Input==5 ]
  Red -> InvalidTransitionState [order 2] : [Input==6 || Input==0]
  Blue -> InvalidTransitionState [order 3] : [Input==6 || Input==0]
  StorageToInit -> InitPosition : after(T_Init_S,sec)
  InitPosition -> InitToStorage [order 1] : [Input==1 || Input==2 || Input==3 || Input==4|| Input==6]
  (default) -> InitPosition
  Red -> RBToYB [order 4] : [Input==2 || Input==1]
  Blue -> RBToYB [order 2] : [Input==1 || Input==2]
  InitPosition -> InitPosition [order 2] : [Input==0]
  Blue -> RBToMixing [order 4] : [Input==5]
  Red -> RBToMixing [order 3] : [Input==5]
  StorageToRB -> (junction 182) [order 2] : [Input==4 &&...
      |  after(T_S_RB,sec)]
  (junction 182) -> Red [order 1] : [blue==0&&red==0]
  StorageToRB -> (junction 179) [order 1] : [Input==3 && after(T_S_RB,sec)]
  (junction 179) -> Blue [order 1] : [blue==0&&red==0]
  Blue -> Red [order 1] : [Input==4]
  Red -> Blue [order 1] : [Input==3]
  data: Input input; invalidTransition output; startMixing output boolean size=1; fillBlack output boolean size=1; fillYellow output boolean size=1; fillBlue output boolean size=1; fillRed output boolean size=1; yellow input; black input; red input; blue input; mixer input; stationError output; T_YB_M constant double =10; T_RB_YB constant double =15; T_RB_M constant double =10; T_S_YB constant double =10; T_S_RB constant double =10; T_YB_RB constant double =15; T_M_S constant double =15; T_Init_S constant double =10

== matlab function FourAGVsFullModel/Subsystem4/MATLAB Function2 ==
  data: u input; y output string
function y= fcn(u)
if(u==1)
    y="station is busy";
else
    y="No Error";
end

== matlab function FourAGVsFullModel/Subsystem5/MATLAB Function3 ==
  data: u input; y output string
function y= fcn(u)
if(u==1)
    y="station is busy";
else
    y="No Error";
end

== matlab function FourAGVsFullModel/Subsystem6/MATLAB Function ==
  data: u input; y output string
function y= fcn(u)
if(u==1)
    y="Invalid Transition";
else
    y="No Error";
end

== matlab function FourAGVsFullModel/Subsystem7/MATLAB Function1 ==
  data: u input; y output string
function y= fcn(u)
if(u==1)
    y="station is busy";
else
    y="No Error";
end
